simulink model "week1problem5"  (R2020a)
settings: Solver=VariableStepAuto  StartTime=0.0  StopTime=10  MaxStep=0.001  RelTol=1e-3
values from neighbouring files (symbols this model uses):
  c = 1e-05    [week1problem5.mat]
  R = 10    [week1problem5.mat]
settings Model: Creator=Admin  LastModifiedBy=Admin

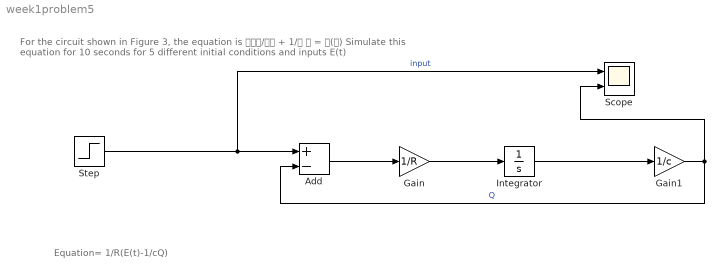
== system week1problem5 ==
  note: Equation= 1/R(E(t)-1/cQ)
  note: For the circuit shown in Figure 3, the equation is 𝑅𝑑𝑄/𝑑𝑡 + 1/𝐶 𝑄 = 𝐸(𝑡)
      | Simulate this equation for 10 seconds for 5 different initial conditions and inputs E(t)
  Add : Sum  Inputs=+-
  Gain : Gain  Gain=1/R
  Gain1 : Gain  Gain=1/c
  Integrator : Integrator
  Scope : Scope  NumInputPorts=2
  Step : Step  SampleTime=0
  wires:
  Add/1 -> Gain/1
  Gain/1 -> Integrator/1
  Integrator/1 -> Gain1/1
  Step/1 -> Scope/1, Add/1  "input"
  Gain1/1 -> Scope/2, Add/2  "Q"
